simulink model "LowpassFilter_Test"  (R2025a)
settings: Solver=FixedStepAuto  StartTime=0.0  StopTime=10.0  RelTol=1e-3
libraries: simulink x1
settings Model: Creator=Polarstern  LastModifiedBy=Polarstern

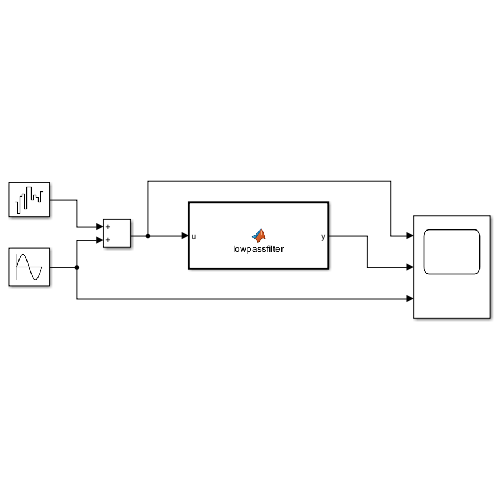
[thumbnail: Simulink's stored preview of the top-level diagram]
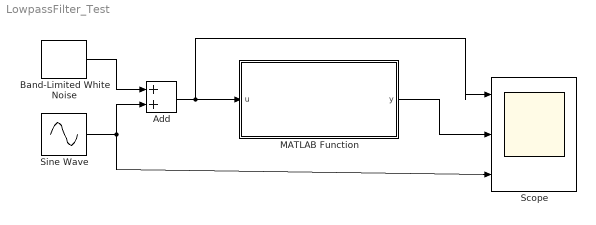
== system LowpassFilter_Test ==
  Add : Sum
  Band-Limited White Noise : simulink/Sources/Band-Limited White Noise  Cov=0.001  Ts=1e-4  seed=[23341]
  MATLAB Function : MATLAB Function  TreatAsAtomicUnit=on
  Scope : Scope  NumInputPorts=3
      settings: ActiveDisplayYMinimum=-18.160384034298193  ActiveDisplayYMaximum=18.578154679859715
  Sine Wave : Sin  Frequency=5  SampleTime=0
  wires:
  Band-Limited White Noise/1 -> Add/1
  Sine Wave/1 -> Scope/3, Add/2
  Add/1 -> Scope/1, MATLAB Function/1(u)
  MATLAB Function/1(y) -> Scope/2

== matlab function LowpassFilter_Test/MATLAB Function ==
  data: u input; y output
function y = lowpassfilter(u)
    %#codegen
    persistent z a b order initialized
    if isempty(initialized)
        initialized = true;
        load_data = load('lpf_params.mat');
        a = load_data.a;
        b = load_data.b;
        order = length(a) - 1;  % Detect order
        z = zeros(order, 1);  % States buffer
    end
    
    % Direct form II transposed
    temp = u;
    for i = 2:length(a)
        temp = temp - a(i) * z(i-1);
    end
    
    y = b(1) * temp;
    for i = 2:length(b)
        y = y + b(i) * z(i-1);
    end
    
    % Update states
    for i = order:-1:2
        z(i) = z(i-1);
    end
    z(1) = temp;

end
